simulink model "TV_2018_HIL"  (R2016a)
settings: Solver=FixedStepAuto  StartTime=0.0  StopTime=inf  FixedStep=0.001  RelTol=1e-3
PreLoadFcn:
  | TV_2017_parameters
values from neighbouring files (symbols this model uses):
  battery_voltage = single(530)    [HIL_parameters.m]    (also in HIL_parameters_2018.m; TV_2017_parameters.m; TV_2017_parameters_VD.m)
  car_params = Simulink_Car_params    [HIL_parameters.m]    (also in HIL_parameters_2018.m; TV_2017_parameters.m; TV_2017_parameters_VD.m)
  i_Diff = 16    [HIL_parameters.m]    (also in HIL_parameters_2018.m; TV_2017_parameters.m)
  Kp = 1    [HIL_parameters.m]    (also in HIL_parameters_2018.m; TV_2017_parameters.m; TV_2017_parameters_VD.m)
  motor_data = struct    [HIL_parameters.m]    (also in HIL_parameters_2018.m; TV_2017_parameters.m)
  powerLimitControl = Simulink_el    [HIL_parameters.m]    (also in HIL_parameters_2018.m; TV_2017_parameters.m; TV_2017_parameters_VD.m)
  settings = Simulink_Settings    [HIL_parameters.m]    (also in HIL_parameters_2018.m; TV_2017_parameters.m; TV_2017_parameters_VD.m)
  SpdC_BCC = 0    [HIL_parameters.m]    (also in HIL_parameters_2018.m; TV_2017_parameters.m; TV_2017_parameters_VD.m)
  Speed_Neg_sat = -21    [HIL_parameters.m]    (also in HIL_parameters_2018.m; TV_2017_parameters.m; TV_2017_parameters_VD.m)
  Speed_Pos_sat = 21    [HIL_parameters.m]    (also in HIL_parameters_2018.m; TV_2017_parameters.m; TV_2017_parameters_VD.m)
  SteeringAngleFL = [-23.80 -22.65 -21.50 -20.34 -19.18 -18.03 -16.86 -15.70 -14.53 -13.35 -12.18 -10.99 -9.80 -8.61 -7.40 -6.19 -4.97 -3.75 -2.51 -1.26 0 1.27 2.56 3.85 5.17 6.50 7.84 9.21 10.59 12.00 13.42 14.88 16.36 17.87 19.41 20.99 22.61 24.26 25.97 27.73 29.54]    [CarSetupAnalysis2018.m]    (also in HIL_parameters_2018.m; TV_2017_parameters.m; TV_2017_parameters_VD.m = [-24.129 -22.950 -21.772 -20.593 -19.413 -18.232 -17.050 -15)
  SteeringAngleFR = [-29.54 -27.73 -25.97 -24.26 -22.61 -20.99 -19.41 -17.87 -16.36 -14.88 -13.42 -12.00 -10.59 -9.21 -7.84 -6.50 -5.17 -3.85 -2.56 -1.27 0 1.26 2.51 3.75 4.97 6.19 7.40 8.61 9.80 10.99 12.18 13.35 14.53 15.70 16.86 18.03 19.18 20.34 21.50 22.65 23.80]    [CarSetupAnalysis2018.m]    (also in HIL_parameters_2018.m; TV_2017_parameters.m; TV_2017_parameters_VD.m = [-29.3050 -27.5340 -25.8140 -24.1410 -22.5110 -20.9180 -19.3)
  SteeringWhAngle = [-105 -99.75 -94.5 -89.25 -84 -78.75 -73.5 -68.25 -63 -57.75 -52.5 -47.25 -42 -36.75 -31.5 -26.25 -21.0 -15.75 -10.5 -5.25 0.0 5.25 10.50 15.75 21.00 26.25 31.50 36.75 42.00 47.25 52.50 57.75  63.00 68.25 73.50 78.75 84.00 89.25 94.50 99.75 105.00]    [TV_2017_parameters_VD.m]
  Tn_n = 0    [HIL_parameters.m]    (also in HIL_parameters_2018.m; TV_2017_parameters.m; TV_2017_parameters_VD.m)
  tractionControl = Simulink_tc    [HIL_parameters.m]    (also in HIL_parameters_2018.m; IterativeTractionControlTuning.m; TV_2017_parameters.m; TV_2017_parameters_VD.m)
  yawMomentGenerator = struct    [HIL_parameters.m]    (also in HIL_parameters_2018.m = Simulink_yawRate2; TV_2017_parameters.m = Simulink_yawRate2)
  yawRateControl = Simulink_yawRate    [HIL_parameters.m]    (also in HIL_parameters_2018.m; TV_2017_parameters.m; TV_2017_parameters_VD.m)
undefined symbols (not defined in the file or in its folder): canChannel, DiscIntNeverNeededParam, magnitude, speedEstimation, TC_Decr_Gas, TC_Derivative, TC_Incr_Gas, TC_On, TC_Relay_Off, TC_Relay_On
libraries: CarMaker4SL x366, simulink_extras x63, canmsglib x55, canlib x41, simulink x37, dspfdesign x2, sldrtlib x1
(part 6 of 15)

== system TV_2018_HIL/CarMaker/Subsystem/Debug Information /Mechanical effect ==
  Gain{8,16..17,19} (4 alike) : Gain  Gain=1/car_params.GR
  Gain{18,20..22} (4 alike) : Gain  Gain=car_params.GR
  Mux7 : Mux
  Pmechanical : Scope
  Product{,1..3} (4 alike) : Product
  Read CM Dict12 : CarMaker4SL/Read CM Dict  xname=Car.WheelSpd_RL  xsync=off
  Read CM Dict13 : CarMaker4SL/Read CM Dict  xname=Car.WheelSpd_FR  xsync=off
  Read CM Dict14 : CarMaker4SL/Read CM Dict  xname=Car.WheelSpd_FL  xsync=off
  Read CM Dict15 : CarMaker4SL/Read CM Dict  xname=PT.WFL.Trq_Drive  xsync=off
  Read CM Dict16 : CarMaker4SL/Read CM Dict  xname=Car.WheelSpd_RR  xsync=off
  Read CM Dict45 : CarMaker4SL/Read CM Dict  xname=PT.WFR.Trq_Drive  xsync=off
  Read CM Dict46 : CarMaker4SL/Read CM Dict  xname=PT.WRL.Trq_Drive  xsync=off
  Read CM Dict47 : CarMaker4SL/Read CM Dict  xname=PT.WRR.Trq_Drive  xsync=off
  To File10 : ToFile  Filename=MAT_files\MechanicalEffect.mat  MatrixName=MechEffect  SaveFormat=Timeseries
  wires:
  Mux7/1 -> Pmechanical/1, To File10/1
  Read CM Dict12/1 -> Gain18/1
  Gain17/1 -> Product1/1
  Read CM Dict14/1 -> Gain22/1
  Gain16/1 -> Product2/1
  Read CM Dict16/1 -> Gain20/1
  Gain19/1 -> Product/1
  Read CM Dict15/1 -> Gain16/1
  Read CM Dict45/1 -> Gain17/1
  Gain8/1 -> Product3/1
  Product1/1 -> Mux7/2  "FR"
  Product/1 -> Mux7/3  "RL"
  Gain22/1 -> Product2/2
  Gain21/1 -> Product1/2
  Read CM Dict47/1 -> Gain8/1
  Product3/1 -> Mux7/4  "RR"
  Read CM Dict13/1 -> Gain21/1
  Gain18/1 -> Product/2
  Gain20/1 -> Product3/2
  Read CM Dict46/1 -> Gain19/1
  Product2/1 -> Mux7/1  "FL"

== system TV_2018_HIL/CarMaker/Subsystem/Debug Information /SA calculation ==
  In1 : Inport
  Bus Selector2 : BusSelector  OutputSignals=steering_wheel_angle
  Degrees to Radians : simulink_extras/Transformations/Degrees to Radians
  Degrees to Radians1 : simulink_extras/Transformations/Degrees to Radians
  FL steer ang lookup deg : Lookup_n-D  NumberOfTableDimensions=1  BreakpointsForDimension1=SteeringAngleFL  Table=SteeringAngleFL  ExtrapMethod=Clip  UseLastTableValue=on  InternalRulePriority=Speed  RndMeth=Simplest  InputSameDT=on
  FR steer ang lookup deg : Lookup_n-D  NumberOfTableDimensions=1  BreakpointsForDimension1=SteeringAngleFR  Table=SteeringAngleFR  ExtrapMethod=Clip  UseLastTableValue=on  InternalRulePriority=Speed  RndMeth=Simplest  InputSameDT=on
  Radians to Degrees1 : simulink_extras/Transformations/Radians to Degrees
  Slip angle calc : MATLAB Function  TreatAsAtomicUnit=on
  Out1 : Outport
  wires:
  Radians to Degrees1/1 -> FL steer ang lookup deg/1, FR steer ang lookup deg/1
  Degrees to Radians1/1 -> Slip angle calc/2(wheel_ang_right)
  Slip angle calc/1(SA) -> Out1/1
  FR steer ang lookup deg/1 -> Degrees to Radians1/1
  Degrees to Radians/1 -> Slip angle calc/1(wheel_ang_left)
  In1/1 -> Slip angle calc/3(sensor), Bus Selector2/1
  FL steer ang lookup deg/1 -> Degrees to Radians/1
  Bus Selector2/1 -> Radians to Degrees1/1  "<steering_wheel_angle>"

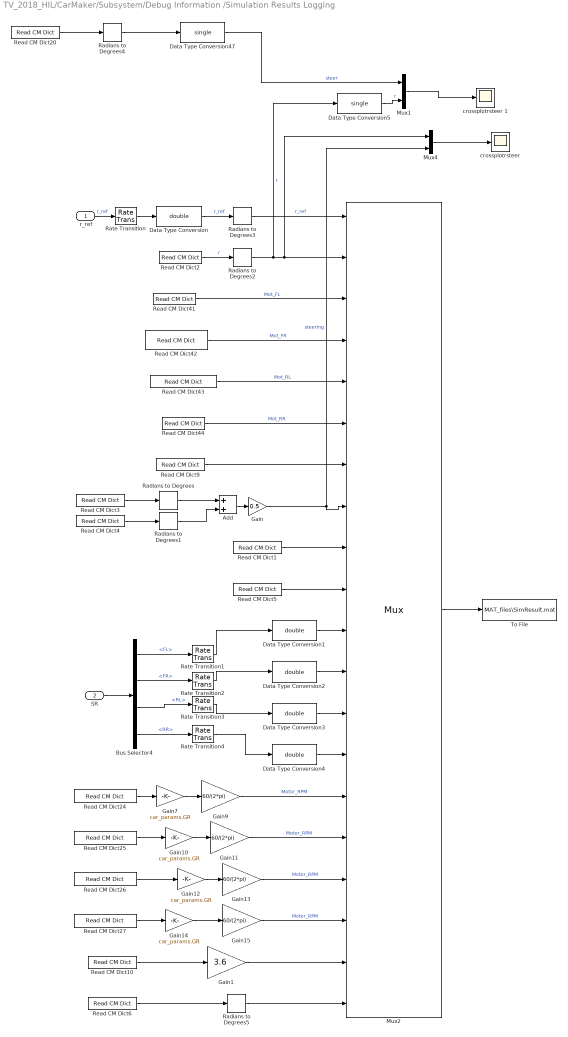
== system TV_2018_HIL/CarMaker/Subsystem/Debug Information /Simulation Results Logging ==
  r_ref : Inport
  SR : Inport  Port=2
  Add : Sum
  Bus Selector4 : BusSelector  OutputSignals=FL,FR,RL,RR
  Data Type Conversion{,1..4} (5 alike) : DataTypeConversion  OutDataTypeStr=double
  Data Type Conversion47 : DataTypeConversion  OutDataTypeStr=single
  Data Type Conversion5 : DataTypeConversion  OutDataTypeStr=single
  Gain : Gain  Gain=0.5
  Gain1 : Gain  Gain=3.6
  Gain{7,10,12,14} (4 alike) : Gain  Gain=car_params.GR
  Gain{9,11,13,15} (4 alike) : Gain  Gain=60/(2*pi)
  Mux1 : Mux  Inputs=2
  Mux2 : Mux  Inputs=20
  Mux4 : Mux  Inputs=2
  Radians to Degrees{,1..5} (6 alike) : simulink_extras/Transformations/Radians to Degrees
  Rate Transition{,1..4} (5 alike) : RateTransition  OutPortSampleTime=0.001
  Read CM Dict1 : CarMaker4SL/Read CM Dict  xname=Vhcl.Fr1.x  xsync=off
  Read CM Dict10 : CarMaker4SL/Read CM Dict  xname=Car.vx  xsync=off
  Read CM Dict2 : CarMaker4SL/Read CM Dict  xname=Car.YawRate  xsync=off
  Read CM Dict20 : CarMaker4SL/Read CM Dict  xname=Vhcl.Steer.Ang  xsync=off
  Read CM Dict24 : CarMaker4SL/Read CM Dict  xname=Car.WheelSpd_FL  xsync=off
  Read CM Dict25 : CarMaker4SL/Read CM Dict  xname=Car.WheelSpd_FR  xsync=off
  Read CM Dict26 : CarMaker4SL/Read CM Dict  xname=Car.WheelSpd_RL  xsync=off
  Read CM Dict27 : CarMaker4SL/Read CM Dict  xname=Car.WheelSpd_RR  xsync=off
  Read CM Dict3 : CarMaker4SL/Read CM Dict  xname=Car.CFR.rz  xsync=off
  Read CM Dict4 : CarMaker4SL/Read CM Dict  xname=Car.CFL.rz  xsync=off
  Read CM Dict41 : CarMaker4SL/Read CM Dict  xname=PT.WFL.Trq_Drive  xsync=off
  Read CM Dict42 : CarMaker4SL/Read CM Dict  xname=PT.WFR.Trq_Drive  xsync=off
  Read CM Dict43 : CarMaker4SL/Read CM Dict  xname=PT.WRL.Trq_Drive  xsync=off
  Read CM Dict44 : CarMaker4SL/Read CM Dict  xname=PT.WRR.Trq_Drive  xsync=off
  Read CM Dict5 : CarMaker4SL/Read CM Dict  xname=Vhcl.Fr1.y  xsync=off
  Read CM Dict6 : CarMaker4SL/Read CM Dict  xname=Vhcl.Steer.Ang  xsync=off
  Read CM Dict9 : CarMaker4SL/Read CM Dict  xname=Car.ay  xsync=off
  To File : ToFile  Filename=MAT_files\SimResult.mat  MatrixName=sim  SaveFormat=Timeseries
  "crossplotrsteer " : Scope
  crossplotrsteer 1 : Scope
  wires:
  r_ref/1 -> Rate Transition/1  "r_ref"
  Read CM Dict2/1 -> Radians to Degrees2/1  "r"
  Data Type Conversion/1 -> Radians to Degrees3/1  "r_ref"
  Read CM Dict42/1 -> Mux2/4  "Mot_FR"
  Read CM Dict43/1 -> Mux2/5  "Mot_RL"
  Read CM Dict41/1 -> Mux2/3  "Mot_FL"
  Read CM Dict44/1 -> Mux2/6  "Mot_RR"
  Read CM Dict9/1 -> Mux2/7
  Read CM Dict3/1 -> Radians to Degrees/1
  Read CM Dict4/1 -> Radians to Degrees1/1
  Radians to Degrees/1 -> Add/1
  Radians to Degrees1/1 -> Add/2
  Radians to Degrees2/1 -> Data Type Conversion5/1, Mux4/1, Mux2/2  "r"
  Radians to Degrees3/1 -> Mux2/1  "r_ref"
  Add/1 -> Gain/1
  Mux2/1 -> To File/1
  Read CM Dict1/1 -> Mux2/9
  Read CM Dict5/1 -> Mux2/10
  Rate Transition/1 -> Data Type Conversion/1
  Mux4/1 -> "crossplotrsteer "/1
  Gain/1 -> Mux2/8, Mux4/2  "steering"
  Bus Selector4/1 -> Rate Transition1/1  "<FL>"
  Bus Selector4/2 -> Rate Transition2/1  "<FR>"
  Bus Selector4/3 -> Rate Transition3/1  "<RL>"
  Bus Selector4/4 -> Rate Transition4/1  "<RR>"
  SR/1 -> Bus Selector4/1
  Rate Transition1/1 -> Data Type Conversion1/1
  Rate Transition2/1 -> Data Type Conversion2/1
  Rate Transition3/1 -> Data Type Conversion3/1
  Rate Transition4/1 -> Data Type Conversion4/1
  Data Type Conversion1/1 -> Mux2/11
  Data Type Conversion2/1 -> Mux2/12
  Data Type Conversion3/1 -> Mux2/13
  Data Type Conversion4/1 -> Mux2/14
  Gain7/1 -> Gain9/1
  Gain9/1 -> Mux2/15  "Motor_RPM"
  Read CM Dict24/1 -> Gain7/1
  Read CM Dict25/1 -> Gain10/1
  Gain10/1 -> Gain11/1
  Gain11/1 -> Mux2/16  "Motor_RPM"
  Gain12/1 -> Gain13/1
  Gain13/1 -> Mux2/17  "Motor_RPM"
  Gain14/1 -> Gain15/1
  Gain15/1 -> Mux2/18  "Motor_RPM"
  Read CM Dict26/1 -> Gain12/1
  Read CM Dict27/1 -> Gain14/1
  Read CM Dict10/1 -> Gain1/1
  Gain1/1 -> Mux2/19
  Read CM Dict20/1 -> Radians to Degrees4/1
  Data Type Conversion47/1 -> Mux1/1  "steer"
  Mux1/1 -> crossplotrsteer 1/1
  Radians to Degrees4/1 -> Data Type Conversion47/1
  Data Type Conversion5/1 -> Mux1/2  "r"
  Read CM Dict6/1 -> Radians to Degrees5/1
  Radians to Degrees5/1 -> Mux2/20

== system TV_2018_HIL/CarMaker/Subsystem/Debug Information /Subsystem ==
  Abs{1..4} (4 alike) : Abs
  Add : Sum  Inputs=++++
  Bus Creator : BusCreator  Inputs=4  OutDataTypeStr=Bus: T_meas
      settings: InheritFromInputs=off
  Bus Creator1 : BusCreator  Inputs=8  OutDataTypeStr=Bus: PowerDebug
      settings: InheritFromInputs=off
  Data Type Conversion{2..5,28..31} (8 alike) : DataTypeConversion  OutDataTypeStr=single
  Divide{,1..3} (4 alike) : Product  Inputs=*/
  Gain{8,16,21..22} (4 alike) : Gain  Gain=1/car_params.GR
  Gain{17,19,23,25} (4 alike) : Gain  Gain=car_params.GR
  Gain{18,20,24,26} (4 alike) : Gain  Gain=60/(2*pi)
  MATLAB Function : MATLAB Function  TreatAsAtomicUnit=on
  Product{,1..3} (4 alike) : Product
  Read CM Dict13 : CarMaker4SL/Read CM Dict  xname=PT.WFL.Trq_Drive  xsync=off
  Read CM Dict14 : CarMaker4SL/Read CM Dict  xname=Car.WheelSpd_FL  xsync=off
  Read CM Dict15 : CarMaker4SL/Read CM Dict  xname=Car.WheelSpd_FR  xsync=off
  Read CM Dict16 : CarMaker4SL/Read CM Dict  xname=Car.WheelSpd_RR  xsync=off
  Read CM Dict45 : CarMaker4SL/Read CM Dict  xname=PT.WFR.Trq_Drive  xsync=off
  Read CM Dict46 : CarMaker4SL/Read CM Dict  xname=PT.WRL.Trq_Drive  xsync=off
  Read CM Dict47 : CarMaker4SL/Read CM Dict  xname=PT.WRR.Trq_Drive  xsync=off
  Read CM Dict50 : CarMaker4SL/Read CM Dict  xname=Car.WheelSpd_RL  xsync=off
  Switch{,1..3} (4 alike) : Switch  Criteria=u2 > Threshold
  motor efficiency table based on RPM and torque : Lookup_n-D  BreakpointsForDimension1=single([1.3,2.7,5.4,7.9,10.4,12.5,14.4,16.0,17.4,18.5,19.6]);  BreakpointsForDimension2=single([500,1000,2000,3000,4000,6000,10000,12000,15000,19000]);  Table=single(reshape([0.6437000036239624,0.5799999833106995,0.44999998807907104,0.3499999940395355,0.28999999165534973,0.23999999463558197,0.20000000298023224,0.17000000178813934,0.14000000059604645,0.12999999523162842,0.10999999940395355,0.7099999785423279,0.699999988079071,0.6100000143051148,0.5099999904632568,0.4399999976158142,0.3799999952316284,0.33000001311302185,0.28999999165534973,0.25,0.2199999988079071,0.20000000298023224,0.7300000190734863,0.7699999809265137,0.7300000190734863,0.6700000166893005,0.6100000143051148,0.550000011920929,0.5,0.44999998807907104,0.4000000059604645,0.36000001430511475,0.33000001311302185,0.7400000095367432,0.800000011920929,0.7900000214576721,0.7400000095367432,0.6899999976158142,0.6399999856948853,0.5899999737739563,0.5400000214576721,0.5,0.46000000834465027,0.41999998688697815,0.75,0.8199999928474426,0.8199999928474426,0.7799999713897705,0.7400000095367432,0.699999988079071,0.6600000262260437,0.6100000143051148,0.5699999928474426,0.5299999713897705,0.49000000953674316,0.7599999904632568,0.8399999737739563,0.8500000238418579,0.8299999833106995,0.800000011920929,0.7699999809265137,0.7400000095367432,0.699999988079071,0.6600000262260437,0.6200000047683716,0.5899999737739563,0.7699999809265137,0.8500000238418579,0.8799999952316284,0.8700000047683716,0.8600000143051148,0.8399999737739563,0.8100000023841858,0.7799999713897705,0.7599999904632568,0.7200000286102295,0.699999988079071,0.7699999809265137,0.8500000238418579,0.8899999856948853,0.8799999952316284,0.8700000047683716,0.8500000238418579,0.8299999833106995,0.8100000023841858,0.7799999713897705,0.7599999904632568,0.7300000190734863,0.7699999809265137,0.8600000143051148,0.8999999761581421,0.8999999761581421,0.8899999856948853,0.8700000047683716,0.8500000238418579,0.8299999833106995,0.8100000023841858,0.7900000214576721,0.6700000166893005,0.7799999713897705,0.8600000143051148,0.8999999761581421,0.9100000262260437,0.8999999761581421,0.8899999856948853,0.8700000047683716,0.8600000143051148,0.8299999833106995,0.7699999809265137,0.699999988079071],11,10));  ExtrapMethod=Clip  UseLastTableValue=on  InternalRulePriority=Speed  RndMeth=Simplest  InputSameDT=on
  motor efficiency table based on RPM and torque 4 : Lookup_n-D  BreakpointsForDimension1=single([1.3,2.7,5.4,7.9,10.4,12.5,14.4,16.0,17.4,18.5,19.6]);  BreakpointsForDimension2=single([500,1000,2000,3000,4000,6000,10000,12000,15000,19000]);  Table=single(reshape([0.6437000036239624,0.5799999833106995,0.44999998807907104,0.3499999940395355,0.28999999165534973,0.23999999463558197,0.20000000298023224,0.17000000178813934,0.14000000059604645,0.12999999523162842,0.10999999940395355,0.7099999785423279,0.699999988079071,0.6100000143051148,0.5099999904632568,0.4399999976158142,0.3799999952316284,0.33000001311302185,0.28999999165534973,0.25,0.2199999988079071,0.20000000298023224,0.7300000190734863,0.7699999809265137,0.7300000190734863,0.6700000166893005,0.6100000143051148,0.550000011920929,0.5,0.44999998807907104,0.4000000059604645,0.36000001430511475,0.33000001311302185,0.7400000095367432,0.800000011920929,0.7900000214576721,0.7400000095367432,0.6899999976158142,0.6399999856948853,0.5899999737739563,0.5400000214576721,0.5,0.46000000834465027,0.41999998688697815,0.75,0.8199999928474426,0.8199999928474426,0.7799999713897705,0.7400000095367432,0.699999988079071,0.6600000262260437,0.6100000143051148,0.5699999928474426,0.5299999713897705,0.49000000953674316,0.7599999904632568,0.8399999737739563,0.8500000238418579,0.8299999833106995,0.800000011920929,0.7699999809265137,0.7400000095367432,0.699999988079071,0.6600000262260437,0.6200000047683716,0.5899999737739563,0.7699999809265137,0.8500000238418579,0.8799999952316284,0.8700000047683716,0.8600000143051148,0.8399999737739563,0.8100000023841858,0.7799999713897705,0.7599999904632568,0.7200000286102295,0.699999988079071,0.7699999809265137,0.8500000238418579,0.8899999856948853,0.8799999952316284,0.8700000047683716,0.8500000238418579,0.8299999833106995,0.8100000023841858,0.7799999713897705,0.7599999904632568,0.7300000190734863,0.7699999809265137,0.8600000143051148,0.8999999761581421,0.8999999761581421,0.8899999856948853,0.8700000047683716,0.8500000238418579,0.8299999833106995,0.8100000023841858,0.7900000214576721,0.6700000166893005,0.7799999713897705,0.8600000143051148,0.8999999761581421,0.9100000262260437,0.8999999761581421,0.8899999856948853,0.8700000047683716,0.8600000143051148,0.8299999833106995,0.7699999809265137,0.699999988079071],11,10));  ExtrapMethod=Clip  UseLastTableValue=on  InternalRulePriority=Speed  RndMeth=Simplest  InputSameDT=on
  motor efficiency table based on RPM and torque2 : Lookup_n-D  BreakpointsForDimension1=single([1.3,2.7,5.4,7.9,10.4,12.5,14.4,16.0,17.4,18.5,19.6]);  BreakpointsForDimension2=single([500,1000,2000,3000,4000,6000,10000,12000,15000,19000]);  Table=single(reshape([0.6437000036239624,0.5799999833106995,0.44999998807907104,0.3499999940395355,0.28999999165534973,0.23999999463558197,0.20000000298023224,0.17000000178813934,0.14000000059604645,0.12999999523162842,0.10999999940395355,0.7099999785423279,0.699999988079071,0.6100000143051148,0.5099999904632568,0.4399999976158142,0.3799999952316284,0.33000001311302185,0.28999999165534973,0.25,0.2199999988079071,0.20000000298023224,0.7300000190734863,0.7699999809265137,0.7300000190734863,0.6700000166893005,0.6100000143051148,0.550000011920929,0.5,0.44999998807907104,0.4000000059604645,0.36000001430511475,0.33000001311302185,0.7400000095367432,0.800000011920929,0.7900000214576721,0.7400000095367432,0.6899999976158142,0.6399999856948853,0.5899999737739563,0.5400000214576721,0.5,0.46000000834465027,0.41999998688697815,0.75,0.8199999928474426,0.8199999928474426,0.7799999713897705,0.7400000095367432,0.699999988079071,0.6600000262260437,0.6100000143051148,0.5699999928474426,0.5299999713897705,0.49000000953674316,0.7599999904632568,0.8399999737739563,0.8500000238418579,0.8299999833106995,0.800000011920929,0.7699999809265137,0.7400000095367432,0.699999988079071,0.6600000262260437,0.6200000047683716,0.5899999737739563,0.7699999809265137,0.8500000238418579,0.8799999952316284,0.8700000047683716,0.8600000143051148,0.8399999737739563,0.8100000023841858,0.7799999713897705,0.7599999904632568,0.7200000286102295,0.699999988079071,0.7699999809265137,0.8500000238418579,0.8899999856948853,0.8799999952316284,0.8700000047683716,0.8500000238418579,0.8299999833106995,0.8100000023841858,0.7799999713897705,0.7599999904632568,0.7300000190734863,0.7699999809265137,0.8600000143051148,0.8999999761581421,0.8999999761581421,0.8899999856948853,0.8700000047683716,0.8500000238418579,0.8299999833106995,0.8100000023841858,0.7900000214576721,0.6700000166893005,0.7799999713897705,0.8600000143051148,0.8999999761581421,0.9100000262260437,0.8999999761581421,0.8899999856948853,0.8700000047683716,0.8600000143051148,0.8299999833106995,0.7699999809265137,0.699999988079071],11,10));  ExtrapMethod=Clip  UseLastTableValue=on  InternalRulePriority=Speed  RndMeth=Simplest  InputSameDT=on
  motor efficiency table based on RPM and torque3 : Lookup_n-D  BreakpointsForDimension1=single([1.3,2.7,5.4,7.9,10.4,12.5,14.4,16.0,17.4,18.5,19.6]);  BreakpointsForDimension2=single([500,1000,2000,3000,4000,6000,10000,12000,15000,19000]);  Table=single(reshape([0.6437000036239624,0.5799999833106995,0.44999998807907104,0.3499999940395355,0.28999999165534973,0.23999999463558197,0.20000000298023224,0.17000000178813934,0.14000000059604645,0.12999999523162842,0.10999999940395355,0.7099999785423279,0.699999988079071,0.6100000143051148,0.5099999904632568,0.4399999976158142,0.3799999952316284,0.33000001311302185,0.28999999165534973,0.25,0.2199999988079071,0.20000000298023224,0.7300000190734863,0.7699999809265137,0.7300000190734863,0.6700000166893005,0.6100000143051148,0.550000011920929,0.5,0.44999998807907104,0.4000000059604645,0.36000001430511475,0.33000001311302185,0.7400000095367432,0.800000011920929,0.7900000214576721,0.7400000095367432,0.6899999976158142,0.6399999856948853,0.5899999737739563,0.5400000214576721,0.5,0.46000000834465027,0.41999998688697815,0.75,0.8199999928474426,0.8199999928474426,0.7799999713897705,0.7400000095367432,0.699999988079071,0.6600000262260437,0.6100000143051148,0.5699999928474426,0.5299999713897705,0.49000000953674316,0.7599999904632568,0.8399999737739563,0.8500000238418579,0.8299999833106995,0.800000011920929,0.7699999809265137,0.7400000095367432,0.699999988079071,0.6600000262260437,0.6200000047683716,0.5899999737739563,0.7699999809265137,0.8500000238418579,0.8799999952316284,0.8700000047683716,0.8600000143051148,0.8399999737739563,0.8100000023841858,0.7799999713897705,0.7599999904632568,0.7200000286102295,0.699999988079071,0.7699999809265137,0.8500000238418579,0.8899999856948853,0.8799999952316284,0.8700000047683716,0.8500000238418579,0.8299999833106995,0.8100000023841858,0.7799999713897705,0.7599999904632568,0.7300000190734863,0.7699999809265137,0.8600000143051148,0.8999999761581421,0.8999999761581421,0.8899999856948853,0.8700000047683716,0.8500000238418579,0.8299999833106995,0.8100000023841858,0.7900000214576721,0.6700000166893005,0.7799999713897705,0.8600000143051148,0.8999999761581421,0.9100000262260437,0.8999999761581421,0.8899999856948853,0.8700000047683716,0.8600000143051148,0.8299999833106995,0.7699999809265137,0.699999988079071],11,10));  ExtrapMethod=Clip  UseLastTableValue=on  InternalRulePriority=Speed  RndMeth=Simplest  InputSameDT=on
  Power debug : Outport
  wires:
  motor efficiency table based on RPM and torque 4/1 -> Product3/2, Divide3/2
  motor efficiency table based on RPM and torque3/1 -> Product2/2, Divide2/2
  Divide1/1 -> Switch1/1
  Product1/1 -> Switch1/3
  MATLAB Function/3(RPM_FL) -> motor efficiency table based on RPM and torque/2
  MATLAB Function/10(Pm_RR) -> Bus Creator1/7, Switch3/2, Product3/1, Divide3/1
  MATLAB Function/2(T_FL) -> Abs1/1
  MATLAB Function/8(T_RL) -> Abs3/1
  Abs4/1 -> motor efficiency table based on RPM and torque 4/1
  Abs2/1 -> motor efficiency table based on RPM and torque2/1
  Data Type Conversion28/1 -> MATLAB Function/1(RPM_FL_IN)
  MATLAB Function/5(T_FR) -> Abs2/1
  MATLAB Function/11(T_RR) -> Abs4/1
  MATLAB Function/12(RPM_RR) -> motor efficiency table based on RPM and torque 4/2
  MATLAB Function/1(Pm_FL) -> Product/1, Switch/2, Divide/1, Bus Creator1/1
  MATLAB Function/7(Pm_RL) -> Switch2/2, Product2/1, Divide2/1, Bus Creator1/5
  Data Type Conversion31/1 -> MATLAB Function/2(RPM_FR_IN)
  Data Type Conversion30/1 -> MATLAB Function/3(RPM_RL_IN)
  Divide/1 -> Switch/1
  Product/1 -> Switch/3
  Data Type Conversion29/1 -> MATLAB Function/4(RPM_RR_IN)
  Bus Creator/1 -> MATLAB Function/5(T)
  motor efficiency table based on RPM and torque/1 -> Divide/2, Product/2
  MATLAB Function/4(Pm_FR) -> Bus Creator1/3, Product1/1, Switch1/2, Divide1/1
  Abs1/1 -> motor efficiency table based on RPM and torque/1
  motor efficiency table based on RPM and torque2/1 -> Divide1/2, Product1/2
  MATLAB Function/6(RPM_FR) -> motor efficiency table based on RPM and torque2/2
  Switch/1 -> Bus Creator1/2, Add/1  "Pe_FL"
  MATLAB Function/9(RPM_RL) -> motor efficiency table based on RPM and torque3/2
  Abs3/1 -> motor efficiency table based on RPM and torque3/1
  Divide2/1 -> Switch2/1
  Divide3/1 -> Switch3/1
  Read CM Dict13/1 -> Gain8/1
  Read CM Dict46/1 -> Gain21/1
  Read CM Dict45/1 -> Gain16/1
  Product3/1 -> Switch3/3
  Switch2/1 -> Bus Creator1/6, Add/3  "Pe_RL"
  Product2/1 -> Switch2/3
  Switch1/1 -> Bus Creator1/4, Add/2  "Pe_FR"
  Switch3/1 -> Add/4, Bus Creator1/8  "Pe_RR"
  Gain24/1 -> Data Type Conversion31/1  "Motor_RPM"
  Read CM Dict15/1 -> Gain23/1
  Gain8/1 -> Data Type Conversion2/1
  Gain22/1 -> Data Type Conversion5/1
  Read CM Dict50/1 -> Gain25/1
  Gain23/1 -> Gain24/1
  Gain19/1 -> Gain20/1
  Bus Creator1/1 -> Power debug/1
  Gain18/1 -> Data Type Conversion29/1  "Motor_RPM"
  Gain26/1 -> Data Type Conversion30/1  "Motor_RPM"
  Read CM Dict14/1 -> Gain19/1
  Data Type Conversion4/1 -> Bus Creator/3  "RL"
  Add/1 -> ?
  Read CM Dict16/1 -> Gain17/1
  Gain17/1 -> Gain18/1
  Data Type Conversion3/1 -> Bus Creator/2  "FR"
  Gain25/1 -> Gain26/1
  Gain16/1 -> Data Type Conversion3/1
  Gain21/1 -> Data Type Conversion4/1
  Data Type Conversion2/1 -> Bus Creator/1  "FL"
  Gain20/1 -> Data Type Conversion28/1  "Motor_RPM"
  Data Type Conversion5/1 -> Bus Creator/4  "RR"
  Read CM Dict47/1 -> Gain22/1

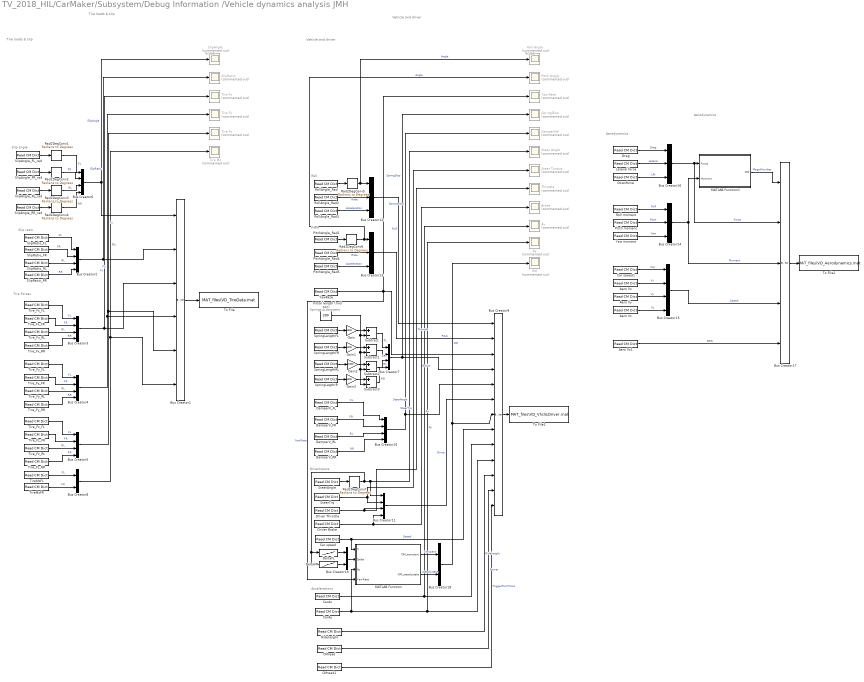
== system TV_2018_HIL/CarMaker/Subsystem/Debug Information /Vehicle dynamics analysis JMH ==
  note: Aerodynamics
  note: Vehicle and driver
  note: Tire loads & slip
  note: Aerodynamics
  note: Tire loads & slip
  note: Vehicle and driver
  note: Tire Forces
  note: Scope
  note: Slip ratio
  note: Slip angle
  note: Scope
  note: Springs & dampers
  note: DriverInputs
  note: Roll
  note: Pitch
  note: Accelerations
  Aero Vx : CarMaker4SL/Read CM Dict  xname=Car.Aero.vres_1.x  xsync=off
  Aero Vy : CarMaker4SL/Read CM Dict  xname=Car.Aero.vres_1.y  xsync=off
  Aero Vz : CarMaker4SL/Read CM Dict  xname=Car.Aero.vres_1.z  xsync=off
  Aero Vz1 : CarMaker4SL/Read CM Dict  xname=DRS  xsync=off
  Ax : Scope  Commented=on
  Ay : Scope  Commented=on
  Brake : Scope  Commented=on
  Bus Creator1 : BusCreator  Inputs=6
  Bus Creator{2..7,10..11,15} (9 alike) : BusCreator  Inputs=4
  Bus Creator{12..14,16} (4 alike) : BusCreator  Inputs=3
  Bus Creator17 : BusCreator  Inputs=5
  Bus Creator18 : BusCreator  Inputs=2
  Bus Creator19 : BusCreator  Inputs=2
  Bus Creator8 : BusCreator  Inputs=2
  Bus Creator9 : BusCreator  Inputs=13
  CMread : CarMaker4SL/Read CM Dict  xname=Power  xsync=off
  CMread1 : CarMaker4SL/Read CM Dict  xname=DM.TriggerPoint.Time  xsync=off
  Car speed : CarMaker4SL/Read CM Dict  xname=Vhcl.v  xsync=off
  Car speed1 : CarMaker4SL/Read CM Dict  xname=Vhcl.v  xsync=off
  CarAx : CarMaker4SL/Read CM Dict  xname=Car.ax  xsync=off
  CarAy : CarMaker4SL/Read CM Dict  xname=Car.ay  xsync=off
  DamperV_FL : CarMaker4SL/Read CM Dict  xname=Car.DampFL.v  xsync=off
  DamperV_FR : CarMaker4SL/Read CM Dict  xname=Car.SpringFR.l  xsync=off
  DamperV_RL : CarMaker4SL/Read CM Dict  xname=Car.SpringRL.l  xsync=off
  DamperV_RR : CarMaker4SL/Read CM Dict  xname=Car.SpringRR.l  xsync=off
  DamperVel : Scope  Commented=on
  DeltaFL : Lookup_n-D  NumberOfTableDimensions=1  BreakpointsForDimension1=SteeringWhAngle  Table=SteeringAngleFL  InterpMethod=Cubic spline  ExtrapMethod=Clip  InternalRulePriority=Speed  RndMeth=Simplest  InputSameDT=on
  DeltaFR : Lookup_n-D  NumberOfTableDimensions=1  BreakpointsForDimension1=SteeringWhAngle  Table=SteeringAngleFR  InterpMethod=Cubic spline  ExtrapMethod=Clip  InternalRulePriority=Speed  RndMeth=Simplest  InputSameDT=on
  Downforce : CarMaker4SL/Read CM Dict  xname=Car.Aero.Frc_1.z  xsync=off
  Drag : CarMaker4SL/Read CM Dict  xname=Car.Aero.Frc_1.x  xsync=off
  Driver Brake : CarMaker4SL/Read CM Dict  xname=DM.Brake  xsync=off
  "Driver Throttle " : CarMaker4SL/Read CM Dict  xname=DM.Gas  xsync=off
  Gain{,1..3} (4 alike) : Gain  Gain=1000
  Initial length (mid pos) : Constant  Value=200
  Lateral force : CarMaker4SL/Read CM Dict  xname=Car.Aero.Frc_1.y  xsync=off
  MATLAB Function : MATLAB Function  TreatAsAtomicUnit=on
  MATLAB Function1 : MATLAB Function  TreatAsAtomicUnit=on
  OM : Scope  Commented=on
  Pitch Angle : Scope  Commented=on
  Pitch moment : CarMaker4SL/Read CM Dict  xname=Car.Aero.Trq_1.y  xsync=off
  PitchAngle_Rad1 : CarMaker4SL/Read CM Dict  xname=Vhcl.Pitch  xsync=off
  PitchAngle_Rad4 : CarMaker4SL/Read CM Dict  xname=Vhcl.PitchVel  xsync=off
  PitchAngle_Rad5 : CarMaker4SL/Read CM Dict  xname=Vhcl.PitchAcc  xsync=off
  Rad2DegConv{1..7} (7 alike) : simulink_extras/Transformations/Radians to Degrees
  Rideheight : CarMaker4SL/Read CM Dict  xname=RideHeight  xsync=off
  Roll Angle : Scope  Commented=on
  Roll moment : CarMaker4SL/Read CM Dict  xname=Car.Aero.Trq_1.x  xsync=off
  RollAngle_Rad : CarMaker4SL/Read CM Dict  xname=Vhcl.Roll  xsync=off
  RollAngle_Rad2 : CarMaker4SL/Read CM Dict  xname=Vhcl.RollVel  xsync=off
  RollAngle_Rad3 : CarMaker4SL/Read CM Dict  xname=Vhcl.RollAcc  xsync=off
  SlipAngle : Scope  Commented=on
  SlipAngle_FL_rad : CarMaker4SL/Read CM Dict  xname=Car.SlipAngleFL  xsync=off
  SlipAngle_FR_rad : CarMaker4SL/Read CM Dict  xname=Car.SlipAngleFR  xsync=off
  SlipAngle_RL_rad : CarMaker4SL/Read CM Dict  xname=Car.SlipAngleRL  xsync=off
  SlipAngle_RR_rad : CarMaker4SL/Read CM Dict  xname=Car.SlipAngleRR  xsync=off
  SlipRatio : Scope  Commented=on
  SlipRatio_FL : CarMaker4SL/Read CM Dict  xname=Car.LongSlipFL  xsync=off
  SlipRatio_FR : CarMaker4SL/Read CM Dict  xname=Car.LongSlipFR  xsync=off
  SlipRatio_RL : CarMaker4SL/Read CM Dict  xname=Car.LongSlipRL  xsync=off
  SlipRatio_RR : CarMaker4SL/Read CM Dict  xname=Car.LongSlipRR  xsync=off
  SpringDisp : Scope  Commented=on
  SpringLegthrR : CarMaker4SL/Read CM Dict  xname=Car.SpringRR.l  xsync=off
  SpringLengthFL : CarMaker4SL/Read CM Dict  xname=Car.SpringFL.l  xsync=off
  SpringLengthFR : CarMaker4SL/Read CM Dict  xname=Car.SpringFR.l  xsync=off
  SpringLengthRL : CarMaker4SL/Read CM Dict  xname=Car.SpringRL.l  xsync=off
  Steer Angle : Scope  Commented=on
  Steer Torque : Scope  Commented=on
  SteerAngle : CarMaker4SL/Read CM Dict  xname=DM.Steer.Ang  xsync=off
  SteerTrq : CarMaker4SL/Read CM Dict  xname=DM.Steer.Trq  xsync=off
  Subtract{,1..3} (4 alike) : Sum  Inputs=+-
  Throttle : Scope  Commented=on
  Tire Fx : Scope  Commented=on
  Tire Fy : Scope  Commented=on
  Tire Fz : Scope  Commented=on
  Tire Mz : Scope  Commented=on
  TireMzFL : CarMaker4SL/Read CM Dict  xname=Car.TrqAlignFL  xsync=off
  TireMzFR : CarMaker4SL/Read CM Dict  xname=Car.TrqAlignFR  xsync=off
  Tire_Fx_FL : CarMaker4SL/Read CM Dict  xname=Car.FxFL  xsync=off
  Tire_Fx_FR : CarMaker4SL/Read CM Dict  xname=Car.FxFR  xsync=off
  Tire_Fx_RL : CarMaker4SL/Read CM Dict  xname=Car.FxRL  xsync=off
  Tire_Fx_RR : CarMaker4SL/Read CM Dict  xname=Car.FxRR  xsync=off
  Tire_Fy_FL : CarMaker4SL/Read CM Dict  xname=Car.FyFL  xsync=off
  Tire_Fy_FR : CarMaker4SL/Read CM Dict  xname=Car.FyFR  xsync=off
  Tire_Fy_RL : CarMaker4SL/Read CM Dict  xname=Car.FyRL  xsync=off
  Tire_Fy_RR : CarMaker4SL/Read CM Dict  xname=Car.FyRR  xsync=off
  Tire_Fz_FL : CarMaker4SL/Read CM Dict  xname=Car.FzFL  xsync=off
  Tire_Fz_FR : CarMaker4SL/Read CM Dict  xname=Car.FzFR  xsync=off
  Tire_Fz_RL : CarMaker4SL/Read CM Dict  xname=Car.FzRL  xsync=off
  Tire_Fz_RR : CarMaker4SL/Read CM Dict  xname=Car.FzRR  xsync=off
  To File : ToFile  Filename=MAT_files\VD_TireData.mat  MatrixName=Tire  SaveFormat=Timeseries
  To File1 : ToFile  Filename=MAT_files\VD_Vhcl&Driver.mat  MatrixName=Vhcl  SaveFormat=Timeseries
  To File2 : ToFile  Filename=MAT_files\VD_Aerodynamics.mat  MatrixName=Aero  SaveFormat=Timeseries
  Yaw Rate : Scope  Commented=on
  Yaw moment : CarMaker4SL/Read CM Dict  xname=Car.Aero.Trq_1.z  xsync=off
  YawRate : CarMaker4SL/Read CM Dict  xname=Car.YawRate  xsync=off
  wires:
  TireMzFR/1 -> Bus Creator8/2  "FR"
  TireMzFL/1 -> Bus Creator8/1  "FL"
  Bus Creator8/1 -> Bus Creator1/6, Tire Mz/1  "Mz"
  Tire_Fx_RR/1 -> Bus Creator3/4  "RR"
  Tire_Fx_RL/1 -> Bus Creator3/3  "RL"
  Rad2DegConv1/1 -> Bus Creator6/1  "FL"
  Rad2DegConv2/1 -> Bus Creator6/2  "FR"
  Bus Creator1/1 -> To File/1
  SlipAngle_RR_rad/1 -> Rad2DegConv4/1
  Tire_Fx_FL/1 -> Bus Creator3/1  "FL"
  Tire_Fy_FR/1 -> Bus Creator4/2  "FR"
  Bus Creator4/1 -> Tire Fy/1, Bus Creator1/4  "Fy"
  Bus Creator5/1 -> Bus Creator1/5, Tire Fz/1  "Fz"
  SlipAngle_RL_rad/1 -> Rad2DegConv3/1
  Tire_Fz_RL/1 -> Bus Creator5/3  "RL"
  Tire_Fz_FL/1 -> Bus Creator5/1  "FL"
  SlipRatio_RL/1 -> Bus Creator2/3  "RL"
  Tire_Fz_FR/1 -> Bus Creator5/2  "FR"
  Tire_Fy_RL/1 -> Bus Creator4/3  "RL"
  Tire_Fy_RR/1 -> Bus Creator4/4  "RR"
  SlipRatio_FR/1 -> Bus Creator2/2  "FR"
  Bus Creator2/1 -> Bus Creator1/2, SlipRatio/1  "SlipRatio"
  SlipAngle_FL_rad/1 -> Rad2DegConv1/1
  Rad2DegConv4/1 -> Bus Creator6/4  "RR"
  SlipAngle_FR_rad/1 -> Rad2DegConv2/1
  Rad2DegConv3/1 -> Bus Creator6/3  "RL"
  Tire_Fz_RR/1 -> Bus Creator5/4  "RR"
  SlipRatio_FL/1 -> Bus Creator2/1  "FL"
  Bus Creator6/1 -> SlipAngle/1, Bus Creator1/1  "SlipAngle"
  SlipRatio_RR/1 -> Bus Creator2/4  "RR"
  Tire_Fx_FR/1 -> Bus Creator3/2  "FR"
  Tire_Fy_FL/1 -> Bus Creator4/1  "FL"
  Bus Creator3/1 -> Bus Creator1/3, Tire Fx/1  "Fx"
  Car speed/1 -> MATLAB Function/1(V), Bus Creator9/8  "Speed"
  MATLAB Function/1(OM_transient) -> Bus Creator18/1  "transient"
  Bus Creator13/1 -> Bus Creator9/2  "Pitch"
  PitchAngle_Rad5/1 -> Bus Creator13/3  "Acceleration"
  PitchAngle_Rad4/1 -> Bus Creator13/2  "Rate"
  RollAngle_Rad3/1 -> Bus Creator12/3  "Acceleration"
  Bus Creator12/1 -> Bus Creator9/1  "Roll"
  RollAngle_Rad2/1 -> Bus Creator12/2  "Rate"
  Subtract3/1 -> Bus Creator7/4  "RR"
  Gain2/1 -> Subtract2/1
  Subtract2/1 -> Bus Creator7/3  "RL"
  Gain1/1 -> Subtract1/1
  Gain/1 -> Subtract/1
  "Driver Throttle "/1 -> Throttle/1, Bus Creator11/3  "Throttle"
  Bus Creator11/1 -> Bus Creator9/6  "Driver"
  Subtract/1 -> Bus Creator7/1  "FL"
  Initial length (mid pos)/1 -> Subtract1/2, Subtract2/2, Subtract3/2, Subtract/2
  RollAngle_Rad/1 -> Rad2DegConv5/1
  Bus Creator7/1 -> Bus Creator9/4, SpringDisp/1  "SpringDisp"
  SpringLengthFL/1 -> Gain/1
  SpringLengthFR/1 -> Gain1/1
  Rad2DegConv5/1 -> Roll Angle/1, Bus Creator12/1  "Angle"
  PitchAngle_Rad1/1 -> Rad2DegConv6/1
  Rad2DegConv6/1 -> Pitch Angle/1, Bus Creator13/1  "Angle"
  SpringLengthRL/1 -> Gain2/1
  Bus Creator9/1 -> To File1/1
  SpringLegthrR/1 -> Gain3/1
  YawRate/1 -> Yaw Rate/1, Bus Creator9/3, MATLAB Function/4(YawRate)  "YawRate"
  DamperV_FR/1 -> Bus Creator10/2  "FR"
  Rad2DegConv7/1 -> DeltaFL/1, DeltaFR/1, Steer Angle/1, Bus Creator11/1  "SteerAngle"
  Driver Brake/1 -> Brake/1, Bus Creator11/4  "Brake"
  SteerTrq/1 -> Steer Torque/1, Bus Creator11/2  "SteerTrq"
  SteerAngle/1 -> Rad2DegConv7/1
  DamperV_FL/1 -> Bus Creator10/1  "FL"
  DamperV_RR/1 -> Bus Creator10/4  "RR"
  DamperV_RL/1 -> Bus Creator10/3  "RL"
  Bus Creator10/1 -> Bus Creator9/5, DamperVel/1  "DamperVel"
  Subtract1/1 -> Bus Creator7/2  "FR"
  Gain3/1 -> Subtract3/1
  Car speed1/1 -> Bus Creator15/1  "Car"
  Bus Creator15/1 -> Bus Creator17/4  "Speed"
  Aero Vz/1 -> Bus Creator15/4  "Vz"
  Aero Vy/1 -> Bus Creator15/3  "Vy"
  Aero Vx/1 -> Bus Creator15/2  "Vx"
  Bus Creator14/1 -> MATLAB Function1/2(Moment), Bus Creator17/3  "Moment"
  Bus Creator16/1 -> MATLAB Function1/1(Force), Bus Creator17/2  "Force"
  MATLAB Function1/1(MM) -> Bus Creator17/1  "MagicMumber"
  Bus Creator17/1 -> To File2/1
  Yaw moment/1 -> Bus Creator14/3  "Yaw"
  Pitch moment/1 -> Bus Creator14/2  "Pitch"
  Roll moment/1 -> Bus Creator14/1  "Roll"
  Downforce/1 -> Bus Creator16/3  "Lift"
  Lateral force/1 -> Bus Creator16/2  "Lateral"
  Drag/1 -> Bus Creator16/1  "Drag"
  CarAx/1 -> Bus Creator9/9, Ax/1  "Ax"
  CarAy/1 -> MATLAB Function/3(Ay), Bus Creator9/10, Ay/1  "Ay"
  MATLAB Function/2(OM_steadystate) -> Bus Creator18/2  "steadystate"
  Bus Creator18/1 -> OM/1, Bus Creator9/7  "OM"
  DeltaFR/1 -> Bus Creator19/2
  DeltaFL/1 -> Bus Creator19/1
  Bus Creator19/1 -> MATLAB Function/2(Delta)
  Aero Vz1/1 -> Bus Creator17/5  "DRS"
  Rideheight/1 -> Bus Creator9/11  "Rideheight"
  CMread/1 -> Bus Creator9/12  "Power"
  CMread1/1 -> Bus Creator9/13  "TriggerPointTime"

== system TV_2018_HIL/CarMaker/Subsystem/Debug Information /add_elements ==
  In1 : Inport
  Demux : Demux
  Sum1 : Sum  Inputs=|++
  Sum2 : Sum  Inputs=|++
  Sum3 : Sum  Inputs=|++
  Out1 : Outport
  wires:
  In1/1 -> Demux/1
  Demux/3 -> Sum3/1
  Demux/4 -> Sum3/2
  Sum3/1 -> Sum2/2
  Sum2/1 -> Sum1/2
  Demux/2 -> Sum2/1
  Demux/1 -> Sum1/1
  Sum1/1 -> Out1/1

== system TV_2018_HIL/CarMaker/Subsystem/Debug Information /addall ==
  In1 : Inport
  Demux : Demux
  Sum : Sum  Inputs=|++
  Sum1 : Sum  Inputs=|++
  Sum2 : Sum  Inputs=|++
  Out1 : Outport
  wires:
  Sum2/1 -> Out1/1
  Demux/1 -> Sum/1
  Sum/1 -> Sum1/1
  Sum1/1 -> Sum2/1
  Demux/2 -> Sum/2
  Demux/3 -> Sum1/2
  Demux/4 -> Sum2/2
  In1/1 -> Demux/1

== system TV_2018_HIL/CarMaker/Subsystem/Debug Information /addall1 ==
  In1 : Inport
  Demux : Demux
  Sum : Sum  Inputs=|++
  Sum1 : Sum  Inputs=|++
  Sum2 : Sum  Inputs=|++
  Out1 : Outport
  wires:
  Sum2/1 -> Out1/1
  Demux/1 -> Sum/1
  Sum/1 -> Sum1/1
  Sum1/1 -> Sum2/1
  Demux/2 -> Sum/2
  Demux/3 -> Sum1/2
  Demux/4 -> Sum2/2
  In1/1 -> Demux/1

== system TV_2018_HIL/CarMaker/Subsystem/Estimations/1st_deriv ==
  signal : Inport
  Diff_Function : MATLAB Function  TreatAsAtomicUnit=on
  Memory : Memory  X0=[0;0;0;0;0;0;0;0;0;0;0;0;0;0;0]  InheritSampleTime=on
  delta_t : Constant  Value=0.01
  deriv : Outport
  deriv1 : Outport  Port=2
  wires:
  delta_t/1 -> Diff_Function/3(delta_t)
  Diff_Function/2(y) -> deriv/1
  signal/1 -> Diff_Function/2(sensors)
  Diff_Function/1(y_old) -> Memory/1
  Memory/1 -> Diff_Function/1("y_old ")
  Diff_Function/3(RPM_der) -> deriv1/1

== system TV_2018_HIL/CarMaker/Subsystem/Estimations/EstimateVx ==
  sensors : Inport
  Fz_est : Inport  Port=2
  velocity_Estimation : MATLAB Function  TreatAsAtomicUnit=on
  v_x_est : Outport
  wires:
  sensors/1 -> velocity_Estimation/1(sensors)
  Fz_est/1 -> velocity_Estimation/2(normalForces)
  velocity_Estimation/1(V_est_x) -> v_x_est/1

== system TV_2018_HIL/CarMaker/Subsystem/Estimations/Fx_Estimation ==
  sensors : Inport
  EstimateFx : MATLAB Function  TreatAsAtomicUnit=on
  T_motor : Outport
  Fx : Outport  Port=2
  wires:
  sensors/1 -> EstimateFx/1(sensors)
  EstimateFx/1(Fx) -> Fx/1
  EstimateFx/2(T_motor) -> T_motor/1

== system TV_2018_HIL/CarMaker/Subsystem/Estimations/Fz_estimators ==
  sensors : Inport
  Fz_Estimation : Subsystem  TreatAsAtomicUnit=on
  Fz_Estimation_acceleration based : Subsystem  TreatAsAtomicUnit=on
  Fz_est_acc : Outport
  Alpha_r_acc : Outport  Port=2
  Fz_est_damp : Outport  Port=3
  Alpha_r_damp : Outport  Port=4
  wires:
  Fz_Estimation_acceleration based/2("alfa_r_acc ") -> Alpha_r_acc/1
  Fz_Estimation/1(Fz_est) -> Fz_est_damp/1
  sensors/1 -> Fz_Estimation_acceleration based/1(sensors), Fz_Estimation/1(sensors)
  Fz_Estimation/2(alfa_r) -> Alpha_r_damp/1
  Fz_Estimation_acceleration based/1("Fz_acc ") -> Fz_est_acc/1

== system TV_2018_HIL/CarMaker/Subsystem/Estimations/RPM_to_linearVelocity ==
  sensors : Inport
  meanWheelAngle : Inport  Port=2
  whl_v_calculation : MATLAB Function  TreatAsAtomicUnit=on
  whl_speed : Outport
  wires:
  whl_v_calculation/1(whl_speed) -> whl_speed/1
  sensors/1 -> whl_v_calculation/1(sensors)
  meanWheelAngle/1 -> whl_v_calculation/2(meanWheelAngle)

== system TV_2018_HIL/CarMaker/Subsystem/Estimations/Subsystem ==
  V_x : Inport
  wheel_v : Inport  Port=2
  Sensors : Inport  Port=3
  SA calculation : Subsystem
  SR_Calculation : Subsystem
  Slip_Detection : Subsystem
  slip : Outport
  SR : Outport  Port=2
  SA : Outport  Port=3
  wires:
  Slip_Detection/1(slip) -> slip/1
  V_x/1 -> SR_Calculation/1(v_x)
  wheel_v/1 -> SR_Calculation/2(whl_v)
  SA calculation/1(SA) -> SA/1
  Sensors/1 -> SA calculation/1(sensor), Slip_Detection/1(sensor), SR_Calculation/3(sensorInput)
  SR_Calculation/1(SR) -> Slip_Detection/2(SR), SR/1

== system TV_2018_HIL/CarMaker/Subsystem/Estimations/calculateMeanWheelAngle ==
  sensorInput : Inport
  calculateWheelangleandSpeed : MATLAB Function  TreatAsAtomicUnit=on
  mean_wheel_angle : Outport
  mean_wheel_speed : Outport  Port=2
  wires:
  sensorInput/1 -> calculateWheelangleandSpeed/1(sensor)
  calculateWheelangleandSpeed/1(mean_wheel_angle) -> mean_wheel_angle/1
  calculateWheelangleandSpeed/2(mean_wheel_speed) -> mean_wheel_speed/1

== system TV_2018_HIL/CarMaker/Subsystem/Estimations/createStateBus ==
  mean_wheel_angle : Inport
  mean_wheel_speed : Inport  Port=2
  Fx : Inport  Port=3
  sensors : Inport  Port=4
  Fz_est : Inport  Port=5
  whl_speed_cog : Inport  Port=6
  SR : Inport  Port=7
  frictionCoefficient : Inport  Port=8
  SA : Inport  Port=9
  v_x : Inport  Port=10
  v_y : Inport  Port=11
  slip : Inport  Port=12
  Bus Creator1 : BusCreator  Inputs=52  OutDataTypeStr=Bus: States  NonVirtualBus=on
      settings: InheritFromInputs=off
  Bus Selector{,2..6} (6 alike) : BusSelector  OutputSignals=FL,FR,RL,RR
  Bus Selector1 : BusSelector  OutputSignals=Input_throttle,Input_brake,KERS_pos,yawRate,yawRate_der,ax,ay,RPM_FL,RPM_FR,RPM_RL,RPM_RR,power,DC_voltage,AMK_motor_temp_FL,AMK_motor_temp_FR,AMK_motor_temp_RL,AMK_motor_temp_RR,AMK_inverter_temp_FL,AMK_inverter_temp_FR,AMK_inverter_temp_RL,AMK_inverter_temp_RR,steering_wheel_angle,steering_wheel_speed
  states : Outport
  wires:
  sensors/1 -> Bus Selector1/1
  Fz_est/1 -> Bus Selector/1
  whl_speed_cog/1 -> Bus Selector2/1
  Fx/1 -> Bus Selector3/1
  SR/1 -> Bus Selector4/1
  Bus Selector1/9 -> Bus Creator1/9  "<RPM_FR>"
  Bus Selector1/8 -> Bus Creator1/8  "<RPM_FL>"
  Bus Selector1/10 -> Bus Creator1/10  "<RPM_RL>"
  Bus Selector1/7 -> Bus Creator1/7  "<ay>"
  Bus Selector1/11 -> Bus Creator1/11  "<RPM_RR>"
  Bus Selector1/6 -> Bus Creator1/6  "<ax>"
  Bus Selector1/12 -> Bus Creator1/12  "<power>"
  Bus Selector1/5 -> Bus Creator1/5  "<yawRate_der>"
  Bus Selector1/13 -> Bus Creator1/13  "<DC_voltage>"
  Bus Selector1/4 -> Bus Creator1/4  "<yawRate>"
  Bus Selector1/3 -> Bus Creator1/3  "<KERS_pos>"
  Bus Selector1/2 -> Bus Creator1/2  "<Input_brake>"
  Bus Selector1/1 -> Bus Creator1/1  "<Input_throttle>"
  mean_wheel_angle/1 -> Bus Creator1/24
  mean_wheel_speed/1 -> Bus Creator1/25
  v_x/1 -> Bus Creator1/26
  v_y/1 -> Bus Creator1/27
  Bus Selector/1 -> Bus Creator1/32  "<FL>"
  Bus Selector/2 -> Bus Creator1/33  "<FR>"
  Bus Selector/3 -> Bus Creator1/34  "<RL>"
  Bus Selector/4 -> Bus Creator1/35  "<RR>"
  Bus Selector2/1 -> Bus Creator1/36  "<FL>"
  Bus Selector2/2 -> Bus Creator1/37  "<FR>"
  Bus Selector2/3 -> Bus Creator1/38  "<RL>"
  Bus Selector2/4 -> Bus Creator1/39  "<RR>"
  Bus Selector4/1 -> Bus Creator1/40  "<FL>"
  Bus Selector4/2 -> Bus Creator1/41  "<FR>"
  Bus Selector4/3 -> Bus Creator1/42  "<RL>"
  Bus Selector4/4 -> Bus Creator1/43  "<RR>"
  Bus Selector3/1 -> Bus Creator1/28  "<FL>"
  Bus Selector3/2 -> Bus Creator1/29  "<FR>"
  Bus Selector3/3 -> Bus Creator1/30  "<RL>"
  Bus Selector3/4 -> Bus Creator1/31  "<RR>"
  frictionCoefficient/1 -> Bus Creator1/52
  Bus Selector1/14 -> Bus Creator1/14  "<AMK_motor_temp_FL>"
  Bus Selector1/15 -> Bus Creator1/15  "<AMK_motor_temp_FR>"
  Bus Selector1/16 -> Bus Creator1/16  "<AMK_motor_temp_RL>"
  Bus Selector1/17 -> Bus Creator1/17  "<AMK_motor_temp_RR>"
  Bus Selector1/18 -> Bus Creator1/18  "<AMK_inverter_temp_FL>"
  Bus Selector1/19 -> Bus Creator1/19  "<AMK_inverter_temp_FR>"
  Bus Selector1/20 -> Bus Creator1/20  "<AMK_inverter_temp_RL>"
  Bus Selector1/21 -> Bus Creator1/21  "<AMK_inverter_temp_RR>"
  SA/1 -> Bus Selector5/1
  Bus Selector5/1 -> Bus Creator1/44  "<FL>"
  Bus Selector5/2 -> Bus Creator1/45  "<FR>"
  Bus Selector5/3 -> Bus Creator1/46  "<RL>"
  Bus Selector5/4 -> Bus Creator1/47  "<RR>"
  Bus Creator1/1 -> states/1
  Bus Selector1/22 -> Bus Creator1/22  "<steering_wheel_angle>"
  Bus Selector1/23 -> Bus Creator1/23  "<steering_wheel_speed>"
  slip/1 -> Bus Selector6/1
  Bus Selector6/1 -> Bus Creator1/48  "<FL>"
  Bus Selector6/2 -> Bus Creator1/49  "<FR>"
  Bus Selector6/3 -> Bus Creator1/50  "<RL>"
  Bus Selector6/4 -> Bus Creator1/51  "<RR>"

== system TV_2018_HIL/CarMaker/Subsystem/Estimations/friction_estimation ==
  Fx : Inport
  SR : Inport  Port=2
  Fz : Inport  Port=3
  estimateFrictionCoefficient : MATLAB Function  TreatAsAtomicUnit=on
  mu : Outport
  mu_estimate : Outport  Port=2
  mu_individual : Outport  Port=3
  normLongTireForce : Outport  Port=4
  wires:
  Fx/1 -> estimateFrictionCoefficient/1(Fx)
  Fz/1 -> estimateFrictionCoefficient/2(Fz)
  SR/1 -> estimateFrictionCoefficient/3(SR)
  estimateFrictionCoefficient/1(mu) -> mu/1
  estimateFrictionCoefficient/3(normLongTireForce) -> normLongTireForce/1
  estimateFrictionCoefficient/2(mu_estimate) -> mu_estimate/1

== system TV_2018_HIL/CarMaker/Subsystem/Estimations/selectVelocity ==
  v_est_x : Inport
  sensors : Inport  Port=2
  Bus Selector : BusSelector  OutputSignals=V_x_INS,V_x_optical
  Bus Selector1 : BusSelector  OutputSignals=V_y_INS,V_y_optical
  Constant1 : Constant  Value=settings.select_velocity_vx
  Constant2 : Constant  Value=settings.select_velocity_vy
  Index Vector : MultiPortSwitch
  Index Vector1 : MultiPortSwitch  DataPortOrder=Specify indices  Inputs=2  DataPortIndices={2,3}
  v_x : Outport
  v_y : Outport  Port=2
  wires:
  Constant1/1 -> Index Vector/1
  v_est_x/1 -> Index Vector/2
  sensors/1 -> Bus Selector1/1, Bus Selector/1
  Bus Selector/1 -> Index Vector/3  "<V_x_INS>"
  Bus Selector/2 -> Index Vector/4  "<V_x_optical>"
  Index Vector/1 -> v_x/1
  Constant2/1 -> Index Vector1/1
  Bus Selector1/1 -> Index Vector1/2  "<V_y_INS>"
  Bus Selector1/2 -> Index Vector1/3  "<V_y_optical>"
  Index Vector1/1 -> v_y/1

== system TV_2018_HIL/CarMaker/IPG Vehicle3/CarAndTrailer/CarAndTrailerUpd/CreateBus Brake.IF.In ==
  In : Inport
  BusCreator : BusCreator  Inputs=9
  Demux : Demux  Outputs=9
  Out : Outport
  wires:
  Demux/9 -> BusCreator/9  "Brake IF Trq_Reg RR"
  Demux/8 -> BusCreator/8  "Brake IF Trq_Reg RL"
  Demux/7 -> BusCreator/7  "Brake IF Trq_Reg FR"
  Demux/6 -> BusCreator/6  "Brake IF Trq_Reg FL"
  Demux/5 -> BusCreator/5  "Brake IF Trq_Reg_max RR"
  Demux/4 -> BusCreator/4  "Brake IF Trq_Reg_max RL"
  Demux/3 -> BusCreator/3  "Brake IF Trq_Reg_max FR"
  Demux/2 -> BusCreator/2  "Brake IF Trq_Reg_max FL"
  Demux/1 -> BusCreator/1  "Brake IF T_env"
  BusCreator/1 -> Out/1
  In/1 -> Demux/1

== system TV_2018_HIL/CarMaker/IPG Vehicle3/CarAndTrailer/Forces/External Suspension Forces ==
  note: The FSpring/FDamp/FStabi/FBuf outputs of this subsystem will be
      | active if the SuspExtFrcs.Kind entry in the vehicle parameter file
      | is either not present or is empty or has the value "CM4SL".
  note: Insert your suspension forces model here.
  Sync_In : Inport
  lSpring : Inport  Port=2
  vDamp : Inport  Port=3
  lStabi : Inport  Port=4
  lBuf : Inport  Port=5
  Bus Creator{,5..7} (4 alike) : BusCreator  Inputs=8
  Bus Creator{1..4} (4 alike) : BusCreator  Inputs=4
  Demux{1..4} (4 alike) : Demux  Outputs=8
  Ground{,1..15} (16 alike) : Ground
  Terminator{1..4,12} (5 alike) : Terminator
  FSpring : Outport
  FDamp : Outport  Port=2
  FStabi : Outport  Port=3
  FBuf : Outport  Port=4
  wires:
  Bus Creator7/1 -> Terminator4/1
  Bus Creator6/1 -> Terminator3/1
  Bus Creator5/1 -> Terminator2/1
  Bus Creator/1 -> Terminator1/1
  Demux4/8 -> Bus Creator7/8  "vBuf RR"
  Demux4/7 -> Bus Creator7/7  "vBuf RL"
  Demux4/6 -> Bus Creator7/6  "vBuf FR"
  Demux4/5 -> Bus Creator7/5  "vBuf FL"
  Demux3/8 -> Bus Creator6/8  "vStabi RR"
  Demux3/7 -> Bus Creator6/7  "vStabi RL"
  Demux3/6 -> Bus Creator6/6  "vStabi FR"
  Demux3/5 -> Bus Creator6/5  "vStabi FL"
  Demux2/8 -> Bus Creator5/8  "vDamp RR"
  Demux2/7 -> Bus Creator5/7  "vDamp RL"
  Demux2/6 -> Bus Creator5/6  "vDamp FR"
  Demux2/5 -> Bus Creator5/5  "vDamp FL"
  Demux1/8 -> Bus Creator/8  "vSpring RR"
  Demux1/7 -> Bus Creator/7  "vSpring RL"
  Demux1/6 -> Bus Creator/6  "vSpring FR"
  Demux1/5 -> Bus Creator/5  "vSpring FL"
  Demux2/4 -> Bus Creator5/4  "lDamp RR"
  Demux2/3 -> Bus Creator5/3  "lDamp RL"
  Demux2/2 -> Bus Creator5/2  "lDamp FR"
  Demux2/1 -> Bus Creator5/1  "lDamp FL"
  Demux1/4 -> Bus Creator/4  "lSpring RR"
  Demux1/3 -> Bus Creator/3  "lSpring RL"
  Demux1/2 -> Bus Creator/2  "lSpring FR"
  Demux1/1 -> Bus Creator/1  "lSpring FL"
  Demux3/4 -> Bus Creator6/4  "lStabi RR"
  Demux3/3 -> Bus Creator6/3  "lStabi RL"
  Demux3/2 -> Bus Creator6/2  "lStabi FR"
  Demux3/1 -> Bus Creator6/1  "lStabi FL"
  lStabi/1 -> Demux3/1
  vDamp/1 -> Demux2/1
  lSpring/1 -> Demux1/1
  Demux4/4 -> Bus Creator7/4  "lBuf RR"
  Demux4/3 -> Bus Creator7/3  "lBuf RL"
  Demux4/2 -> Bus Creator7/2  "lBuf FR"
  Demux4/1 -> Bus Creator7/1  "lBuf FL"
  lBuf/1 -> Demux4/1
  Ground14/1 -> Bus Creator4/1  "FBuf FL"
  Ground15/1 -> Bus Creator4/2  "FBuf FR"
  Ground12/1 -> Bus Creator4/3  "FBuf RL"
  Ground13/1 -> Bus Creator4/4  "FBuf RR"
  Bus Creator4/1 -> FBuf/1
  Sync_In/1 -> Terminator12/1
  Bus Creator2/1 -> FSpring/1
  Ground/1 -> Bus Creator2/1  "FSpring FL"
  Ground1/1 -> Bus Creator2/2  "FSpring FR"
  Ground2/1 -> Bus Creator2/3  "FSpring RL"
  Ground3/1 -> Bus Creator2/4  "FSpring RR"
  Ground4/1 -> Bus Creator1/1  "FDamp FL"
  Ground5/1 -> Bus Creator1/2  "FDamp FR"
  Ground6/1 -> Bus Creator1/3  "FDamp RL"
  Ground7/1 -> Bus Creator1/4  "FDamp RR"
  Bus Creator1/1 -> FDamp/1
  Ground8/1 -> Bus Creator3/1  "FStabi FL"
  Ground9/1 -> Bus Creator3/2  "FStabi FR"
  Ground10/1 -> Bus Creator3/3  "FStabi RL"
  Ground11/1 -> Bus Creator3/4  "FStabi RR"
  Bus Creator3/1 -> FStabi/1
